simulink model "Charge_1_V1_experiment"  (R2018b)
settings: Solver=FixedStepDiscrete  StartTime=0.0  StopTime=1  FixedStep=0.001  RelTol=1e-3
PreLoadFcn:
  | librarySetup
  | eval([bdroot,'_startup']) %Calling [modelName]_startup.m
undefined symbols (not defined in the file or in its folder): A0, A1, Car1__Authorize, Car2_Authorize, CON2, CON3, CON4, Control_Mode_In, CurrentSP, D10, D12, D13, D2, D3, D4, D5, D6, D7, D8, Free_Charge, Frequency_High_Point, Frequency_Low_Point, Frequency_Mid_high, Frequency_Mid_low, HVol_High_Point, HVol_Low_Point, HVol_Mid_high, HVol_Mid_low, HVoltage_Factor, SeconCar_ThreePhase, V_Current_five, V_Current_four, V_Current_one, V_Current_six, V_Current_three, V_Current_two, V_Frequency, V_MaxPliot, V_MinPliot, Vol_High_Point, Vol_Low_Point, Vol_Mid_high, Vol_Mid_low, Voltage_Factor, Voltage_Mode_Test
libraries: simulink x324, HANcoder_STM32_Target x30, powerlib_meascontrol x8, simulink_extras x2
(part 8 of 13)

== system Charge_1_V1_experiment/HANcoder STM32 Target - E407-STM32 algorithm/Energy Meter/Energymeter_Request/RequestMessages_Enable /Subsystem ==
  In1 : Inport
  Compare To Constant11 : simulink/Logic and Bit Operations/Compare To Constant  relop=<=  const=15  OutDataTypeStr=boolean
  Compare To Constant9 : simulink/Logic and Bit Operations/Compare To Constant  relop=>=  const=0  OutDataTypeStr=boolean
  Logical Operator : Logic  AllPortsSameDT=off  OutDataTypeStr=boolean
  Out1 : Outport
  wires:
  Logical Operator/1 -> Out1/1
  Compare To Constant9/1 -> Logical Operator/1
  Compare To Constant11/1 -> Logical Operator/2
  In1/1 -> Compare To Constant11/1, Compare To Constant9/1

== system Charge_1_V1_experiment/HANcoder STM32 Target - E407-STM32 algorithm/Energy Meter/Energymeter_Request/RequestMessages_Enable /Subsystem1 ==
  In1 : Inport
  Compare To Constant19 : simulink/Logic and Bit Operations/Compare To Constant  relop=>=  const=200  OutDataTypeStr=boolean
  Compare To Constant20 : simulink/Logic and Bit Operations/Compare To Constant  relop=<=  const=215  OutDataTypeStr=boolean
  Logical Operator2 : Logic  AllPortsSameDT=off  OutDataTypeStr=boolean
  Out1 : Outport
  wires:
  In1/1 -> Compare To Constant20/1, Compare To Constant19/1
  Compare To Constant19/1 -> Logical Operator2/1
  Compare To Constant20/1 -> Logical Operator2/2
  Logical Operator2/1 -> Out1/1

== system Charge_1_V1_experiment/HANcoder STM32 Target - E407-STM32 algorithm/Energy Meter/Energymeter_Request/RequestMessages_Enable /Subsystem2 ==
  In1 : Inport
  Compare To Constant19 : simulink/Logic and Bit Operations/Compare To Constant  relop=>=  const=400  OutDataTypeStr=boolean
  Compare To Constant20 : simulink/Logic and Bit Operations/Compare To Constant  relop=<=  const=415  OutDataTypeStr=boolean
  Logical Operator2 : Logic  AllPortsSameDT=off  OutDataTypeStr=boolean
  Out1 : Outport
  wires:
  Logical Operator2/1 -> Out1/1
  Compare To Constant20/1 -> Logical Operator2/2
  Compare To Constant19/1 -> Logical Operator2/1
  In1/1 -> Compare To Constant19/1, Compare To Constant20/1

== system Charge_1_V1_experiment/HANcoder STM32 Target - E407-STM32 algorithm/Energy Meter/Energymeter_Request/RequestMessages_Enable /Subsystem3 ==
  In1 : Inport
  Compare To Constant19 : simulink/Logic and Bit Operations/Compare To Constant  relop=>=  const=600  OutDataTypeStr=boolean
  Compare To Constant20 : simulink/Logic and Bit Operations/Compare To Constant  relop=<=  const=615  OutDataTypeStr=boolean
  Logical Operator2 : Logic  AllPortsSameDT=off  OutDataTypeStr=boolean
  Out1 : Outport
  wires:
  In1/1 -> Compare To Constant20/1, Compare To Constant19/1
  Compare To Constant19/1 -> Logical Operator2/1
  Compare To Constant20/1 -> Logical Operator2/2
  Logical Operator2/1 -> Out1/1

== system Charge_1_V1_experiment/HANcoder STM32 Target - E407-STM32 algorithm/Energy Meter/Energymeter_Request/RequestMessages_Enable /Subsystem4 ==
  In1 : Inport
  Compare To Constant19 : simulink/Logic and Bit Operations/Compare To Constant  relop=>=  const=800  OutDataTypeStr=boolean
  Compare To Constant20 : simulink/Logic and Bit Operations/Compare To Constant  relop=<=  const=815  OutDataTypeStr=boolean
  Logical Operator2 : Logic  AllPortsSameDT=off  OutDataTypeStr=boolean
  Out1 : Outport
  wires:
  Logical Operator2/1 -> Out1/1
  Compare To Constant20/1 -> Logical Operator2/2
  Compare To Constant19/1 -> Logical Operator2/1
  In1/1 -> Compare To Constant19/1, Compare To Constant20/1

== system Charge_1_V1_experiment/HANcoder STM32 Target - E407-STM32 algorithm/Energy Meter/Energymeter_Request/Voltage_meter_1/Read_Gyro1 ==
  note: 01040000000271CB
  Trigger : TriggerPort  VariantControl=Variant
  Constant : Constant  Value=hex2dec('01')  OutDataTypeStr=uint8  SampleTime=-1
  UART send : Subsystem  Tag=HANcoder_TARGET_STM32_E407  AncestorBlock=HANcoder_STM32_Target/STM32-E407/UART/UART send  mask(UART send){channel=UART2: CON PD - 8 & 9, useStatusOut=off, tsamp=-1}
      mask prompts: useStatusOut "Use status outport"; tsamp "Sample time"
      mask help:
      | Function
      | ==========
      | Transmits a byte on the UART communication interface.
      |
      | Parameters per channel
      | ======================
      | - Select channel (TX & RX)
      | - Select if the status output should be enabled.
      |
      | Inputs
      | ======
      | - The byte to send
      |
      | Outputs
      | =======
      | - When the status output is 0, the byte could not be transmitted. Probably
      |   because the transmit buffer was configured too small.
      mask init:
      | uartChannelInfoStr = sfcn_uart_send_mcb(2, channel, useStatusOut);
      settings: MoveFcn=drawLogos
      mask Help: web('sfcn_uart_send.html')
      mask TypeOptions channel: UART1: CON3 - D1 & D0 | UART2: CON PD - 8 & 9 | UART3: CON PD - 11 & 12 | UART6: UEXT - 3 & 4
      mask Display: fprintf('UART send\n%s', uartChannelInfoStr);patch([245 251 251],[8 14 2],[1 0 0]);patch([253 253 259],[14 2 8],[0 0 0.35]);
  wires:
  Constant/1 -> UART send/1(In1)

== system Charge_1_V1_experiment/HANcoder STM32 Target - E407-STM32 algorithm/Energy Meter/Energymeter_Request/Voltage_meter_1/Read_Gyro2 ==
  note: 01040000000271CB
  Trigger : TriggerPort  VariantControl=Variant
  Constant1 : Constant  Value=hex2dec('04')  OutDataTypeStr=uint8  SampleTime=-1
  UART send : Subsystem  Tag=HANcoder_TARGET_STM32_E407  AncestorBlock=HANcoder_STM32_Target/STM32-E407/UART/UART send  mask(UART send){channel=UART2: CON PD - 8 & 9, useStatusOut=off, tsamp=-1}
      mask prompts: useStatusOut "Use status outport"; tsamp "Sample time"
      mask help:
      | Function
      | ==========
      | Transmits a byte on the UART communication interface.
      |
      | Parameters per channel
      | ======================
      | - Select channel (TX & RX)
      | - Select if the status output should be enabled.
      |
      | Inputs
      | ======
      | - The byte to send
      |
      | Outputs
      | =======
      | - When the status output is 0, the byte could not be transmitted. Probably
      |   because the transmit buffer was configured too small.
      mask init:
      | uartChannelInfoStr = sfcn_uart_send_mcb(2, channel, useStatusOut);
      settings: MoveFcn=drawLogos
      mask Help: web('sfcn_uart_send.html')
      mask TypeOptions channel: UART1: CON3 - D1 & D0 | UART2: CON PD - 8 & 9 | UART3: CON PD - 11 & 12 | UART6: UEXT - 3 & 4
      mask Display: fprintf('UART send\n%s', uartChannelInfoStr);patch([245 251 251],[8 14 2],[1 0 0]);patch([253 253 259],[14 2 8],[0 0 0.35]);
  wires:
  Constant1/1 -> UART send/1(In1)

== system Charge_1_V1_experiment/HANcoder STM32 Target - E407-STM32 algorithm/Energy Meter/Energymeter_Request/Voltage_meter_1/Read_Gyro3 ==
  note: 01040000000271CB
  Trigger : TriggerPort  VariantControl=Variant
  Constant2 : Constant  Value=hex2dec('00')  OutDataTypeStr=uint8  SampleTime=-1
  UART send : Subsystem  Tag=HANcoder_TARGET_STM32_E407  AncestorBlock=HANcoder_STM32_Target/STM32-E407/UART/UART send  mask(UART send){channel=UART2: CON PD - 8 & 9, useStatusOut=off, tsamp=-1}
      mask prompts: useStatusOut "Use status outport"; tsamp "Sample time"
      mask help:
      | Function
      | ==========
      | Transmits a byte on the UART communication interface.
      |
      | Parameters per channel
      | ======================
      | - Select channel (TX & RX)
      | - Select if the status output should be enabled.
      |
      | Inputs
      | ======
      | - The byte to send
      |
      | Outputs
      | =======
      | - When the status output is 0, the byte could not be transmitted. Probably
      |   because the transmit buffer was configured too small.
      mask init:
      | uartChannelInfoStr = sfcn_uart_send_mcb(2, channel, useStatusOut);
      settings: MoveFcn=drawLogos
      mask Help: web('sfcn_uart_send.html')
      mask TypeOptions channel: UART1: CON3 - D1 & D0 | UART2: CON PD - 8 & 9 | UART3: CON PD - 11 & 12 | UART6: UEXT - 3 & 4
      mask Display: fprintf('UART send\n%s', uartChannelInfoStr);patch([245 251 251],[8 14 2],[1 0 0]);patch([253 253 259],[14 2 8],[0 0 0.35]);
  wires:
  Constant2/1 -> UART send/1(In1)

== system Charge_1_V1_experiment/HANcoder STM32 Target - E407-STM32 algorithm/Energy Meter/Energymeter_Request/Voltage_meter_1/Read_Gyro4 ==
  note: 01040000000271CB
  Trigger : TriggerPort  VariantControl=Variant
  Constant4 : Constant  Value=hex2dec('00')  OutDataTypeStr=uint8  SampleTime=-1
  UART send : Subsystem  Tag=HANcoder_TARGET_STM32_E407  AncestorBlock=HANcoder_STM32_Target/STM32-E407/UART/UART send  mask(UART send){channel=UART2: CON PD - 8 & 9, useStatusOut=off, tsamp=-1}
      mask prompts: useStatusOut "Use status outport"; tsamp "Sample time"
      mask help:
      | Function
      | ==========
      | Transmits a byte on the UART communication interface.
      |
      | Parameters per channel
      | ======================
      | - Select channel (TX & RX)
      | - Select if the status output should be enabled.
      |
      | Inputs
      | ======
      | - The byte to send
      |
      | Outputs
      | =======
      | - When the status output is 0, the byte could not be transmitted. Probably
      |   because the transmit buffer was configured too small.
      mask init:
      | uartChannelInfoStr = sfcn_uart_send_mcb(2, channel, useStatusOut);
      settings: MoveFcn=drawLogos
      mask Help: web('sfcn_uart_send.html')
      mask TypeOptions channel: UART1: CON3 - D1 & D0 | UART2: CON PD - 8 & 9 | UART3: CON PD - 11 & 12 | UART6: UEXT - 3 & 4
      mask Display: fprintf('UART send\n%s', uartChannelInfoStr);patch([245 251 251],[8 14 2],[1 0 0]);patch([253 253 259],[14 2 8],[0 0 0.35]);
  wires:
  Constant4/1 -> UART send/1(In1)

== system Charge_1_V1_experiment/HANcoder STM32 Target - E407-STM32 algorithm/Energy Meter/Energymeter_Request/Voltage_meter_1/Read_Gyro5 ==
  note: 01040000000271CB
  Trigger : TriggerPort  VariantControl=Variant
  Constant5 : Constant  Value=hex2dec('00')  OutDataTypeStr=uint8  SampleTime=-1
  UART send : Subsystem  Tag=HANcoder_TARGET_STM32_E407  AncestorBlock=HANcoder_STM32_Target/STM32-E407/UART/UART send  mask(UART send){channel=UART2: CON PD - 8 & 9, useStatusOut=off, tsamp=-1}
      mask prompts: useStatusOut "Use status outport"; tsamp "Sample time"
      mask help:
      | Function
      | ==========
      | Transmits a byte on the UART communication interface.
      |
      | Parameters per channel
      | ======================
      | - Select channel (TX & RX)
      | - Select if the status output should be enabled.
      |
      | Inputs
      | ======
      | - The byte to send
      |
      | Outputs
      | =======
      | - When the status output is 0, the byte could not be transmitted. Probably
      |   because the transmit buffer was configured too small.
      mask init:
      | uartChannelInfoStr = sfcn_uart_send_mcb(2, channel, useStatusOut);
      settings: MoveFcn=drawLogos
      mask Help: web('sfcn_uart_send.html')
      mask TypeOptions channel: UART1: CON3 - D1 & D0 | UART2: CON PD - 8 & 9 | UART3: CON PD - 11 & 12 | UART6: UEXT - 3 & 4
      mask Display: fprintf('UART send\n%s', uartChannelInfoStr);patch([245 251 251],[8 14 2],[1 0 0]);patch([253 253 259],[14 2 8],[0 0 0.35]);
  wires:
  Constant5/1 -> UART send/1(In1)

== system Charge_1_V1_experiment/HANcoder STM32 Target - E407-STM32 algorithm/Energy Meter/Energymeter_Request/Voltage_meter_1/Read_Gyro6 ==
  note: 01040000000271CB
  Trigger : TriggerPort  VariantControl=Variant
  Constant6 : Constant  Value=hex2dec('06')  OutDataTypeStr=uint8  SampleTime=-1
  Terminator2 : Terminator
  UART send : Subsystem  Tag=HANcoder_TARGET_STM32_E407  AncestorBlock=HANcoder_STM32_Target/STM32-E407/UART/UART send  mask(UART send){channel=UART2: CON PD - 8 & 9, useStatusOut=off, tsamp=-1}
      mask prompts: useStatusOut "Use status outport"; tsamp "Sample time"
      mask help:
      | Function
      | ==========
      | Transmits a byte on the UART communication interface.
      |
      | Parameters per channel
      | ======================
      | - Select channel (TX & RX)
      | - Select if the status output should be enabled.
      |
      | Inputs
      | ======
      | - The byte to send
      |
      | Outputs
      | =======
      | - When the status output is 0, the byte could not be transmitted. Probably
      |   because the transmit buffer was configured too small.
      mask init:
      | uartChannelInfoStr = sfcn_uart_send_mcb(2, channel, useStatusOut);
      settings: MoveFcn=drawLogos
      mask Help: web('sfcn_uart_send.html')
      mask TypeOptions channel: UART1: CON3 - D1 & D0 | UART2: CON PD - 8 & 9 | UART3: CON PD - 11 & 12 | UART6: UEXT - 3 & 4
      mask Display: fprintf('UART send\n%s', uartChannelInfoStr);patch([245 251 251],[8 14 2],[1 0 0]);patch([253 253 259],[14 2 8],[0 0 0.35]);
  wires:
  Constant6/1 -> UART send/1(In1)

== system Charge_1_V1_experiment/HANcoder STM32 Target - E407-STM32 algorithm/Energy Meter/Energymeter_Request/Voltage_meter_1/Read_Gyro7 ==
  note: 01040000000271CB
  Trigger : TriggerPort  VariantControl=Variant
  Constant1 : Constant  Value=hex2dec('71')  OutDataTypeStr=uint8  SampleTime=-1
  Constant3 : Constant  Value=hex2dec('70')  OutDataTypeStr=uint8  SampleTime=-1
  UART send : Subsystem  Tag=HANcoder_TARGET_STM32_E407  AncestorBlock=HANcoder_STM32_Target/STM32-E407/UART/UART send  mask(UART send){channel=UART2: CON PD - 8 & 9, useStatusOut=off, tsamp=-1}
      mask prompts: useStatusOut "Use status outport"; tsamp "Sample time"
      mask help:
      | Function
      | ==========
      | Transmits a byte on the UART communication interface.
      |
      | Parameters per channel
      | ======================
      | - Select channel (TX & RX)
      | - Select if the status output should be enabled.
      |
      | Inputs
      | ======
      | - The byte to send
      |
      | Outputs
      | =======
      | - When the status output is 0, the byte could not be transmitted. Probably
      |   because the transmit buffer was configured too small.
      mask init:
      | uartChannelInfoStr = sfcn_uart_send_mcb(2, channel, useStatusOut);
      settings: MoveFcn=drawLogos
      mask Help: web('sfcn_uart_send.html')
      mask TypeOptions channel: UART1: CON3 - D1 & D0 | UART2: CON PD - 8 & 9 | UART3: CON PD - 11 & 12 | UART6: UEXT - 3 & 4
      mask Display: fprintf('UART send\n%s', uartChannelInfoStr);patch([245 251 251],[8 14 2],[1 0 0]);patch([253 253 259],[14 2 8],[0 0 0.35]);
  wires:
  Constant3/1 -> UART send/1(In1)

== system Charge_1_V1_experiment/HANcoder STM32 Target - E407-STM32 algorithm/Energy Meter/Energymeter_Request/Voltage_meter_1/Read_Gyro8 ==
  note: 01040000000271CB
  Trigger : TriggerPort  VariantControl=Variant
  Constant1 : Constant  Value=hex2dec('CB')  OutDataTypeStr=uint8  SampleTime=-1
  Constant7 : Constant  Value=hex2dec('08')  OutDataTypeStr=uint8  SampleTime=-1
  UART send : Subsystem  Tag=HANcoder_TARGET_STM32_E407  AncestorBlock=HANcoder_STM32_Target/STM32-E407/UART/UART send  mask(UART send){channel=UART2: CON PD - 8 & 9, useStatusOut=off, tsamp=-1}
      mask prompts: useStatusOut "Use status outport"; tsamp "Sample time"
      mask help:
      | Function
      | ==========
      | Transmits a byte on the UART communication interface.
      |
      | Parameters per channel
      | ======================
      | - Select channel (TX & RX)
      | - Select if the status output should be enabled.
      |
      | Inputs
      | ======
      | - The byte to send
      |
      | Outputs
      | =======
      | - When the status output is 0, the byte could not be transmitted. Probably
      |   because the transmit buffer was configured too small.
      mask init:
      | uartChannelInfoStr = sfcn_uart_send_mcb(2, channel, useStatusOut);
      settings: MoveFcn=drawLogos
      mask Help: web('sfcn_uart_send.html')
      mask TypeOptions channel: UART1: CON3 - D1 & D0 | UART2: CON PD - 8 & 9 | UART3: CON PD - 11 & 12 | UART6: UEXT - 3 & 4
      mask Display: fprintf('UART send\n%s', uartChannelInfoStr);patch([245 251 251],[8 14 2],[1 0 0]);patch([253 253 259],[14 2 8],[0 0 0.35]);
  wires:
  Constant7/1 -> UART send/1(In1)

== system Charge_1_V1_experiment/HANcoder STM32 Target - E407-STM32 algorithm/Energy Meter/Energymeter_Request/Voltage_meter_2/Read_Gyro1 ==
  note: 01040000000271CB
  Trigger : TriggerPort  VariantControl=Variant
  Constant : Constant  Value=hex2dec('02')  OutDataTypeStr=uint8  SampleTime=-1
  UART send : Subsystem  Tag=HANcoder_TARGET_STM32_E407  AncestorBlock=HANcoder_STM32_Target/STM32-E407/UART/UART send  mask(UART send){channel=UART2: CON PD - 8 & 9, useStatusOut=off, tsamp=-1}
      mask prompts: useStatusOut "Use status outport"; tsamp "Sample time"
      mask help:
      | Function
      | ==========
      | Transmits a byte on the UART communication interface.
      |
      | Parameters per channel
      | ======================
      | - Select channel (TX & RX)
      | - Select if the status output should be enabled.
      |
      | Inputs
      | ======
      | - The byte to send
      |
      | Outputs
      | =======
      | - When the status output is 0, the byte could not be transmitted. Probably
      |   because the transmit buffer was configured too small.
      mask init:
      | uartChannelInfoStr = sfcn_uart_send_mcb(2, channel, useStatusOut);
      settings: MoveFcn=drawLogos
      mask Help: web('sfcn_uart_send.html')
      mask TypeOptions channel: UART1: CON3 - D1 & D0 | UART2: CON PD - 8 & 9 | UART3: CON PD - 11 & 12 | UART6: UEXT - 3 & 4
      mask Display: fprintf('UART send\n%s', uartChannelInfoStr);patch([245 251 251],[8 14 2],[1 0 0]);patch([253 253 259],[14 2 8],[0 0 0.35]);
  wires:
  Constant/1 -> UART send/1(In1)

== system Charge_1_V1_experiment/HANcoder STM32 Target - E407-STM32 algorithm/Energy Meter/Energymeter_Request/Voltage_meter_2/Read_Gyro2 ==
  note: 01040000000271CB
  Trigger : TriggerPort  VariantControl=Variant
  Constant1 : Constant  Value=hex2dec('04')  OutDataTypeStr=uint8  SampleTime=-1
  UART send : Subsystem  Tag=HANcoder_TARGET_STM32_E407  AncestorBlock=HANcoder_STM32_Target/STM32-E407/UART/UART send  mask(UART send){channel=UART2: CON PD - 8 & 9, useStatusOut=off, tsamp=-1}
      mask prompts: useStatusOut "Use status outport"; tsamp "Sample time"
      mask help:
      | Function
      | ==========
      | Transmits a byte on the UART communication interface.
      |
      | Parameters per channel
      | ======================
      | - Select channel (TX & RX)
      | - Select if the status output should be enabled.
      |
      | Inputs
      | ======
      | - The byte to send
      |
      | Outputs
      | =======
      | - When the status output is 0, the byte could not be transmitted. Probably
      |   because the transmit buffer was configured too small.
      mask init:
      | uartChannelInfoStr = sfcn_uart_send_mcb(2, channel, useStatusOut);
      settings: MoveFcn=drawLogos
      mask Help: web('sfcn_uart_send.html')
      mask TypeOptions channel: UART1: CON3 - D1 & D0 | UART2: CON PD - 8 & 9 | UART3: CON PD - 11 & 12 | UART6: UEXT - 3 & 4
      mask Display: fprintf('UART send\n%s', uartChannelInfoStr);patch([245 251 251],[8 14 2],[1 0 0]);patch([253 253 259],[14 2 8],[0 0 0.35]);
  wires:
  Constant1/1 -> UART send/1(In1)

== system Charge_1_V1_experiment/HANcoder STM32 Target - E407-STM32 algorithm/Energy Meter/Energymeter_Request/Voltage_meter_2/Read_Gyro3 ==
  note: 01040000000271CB
  Trigger : TriggerPort  VariantControl=Variant
  Constant2 : Constant  Value=hex2dec('00')  OutDataTypeStr=uint8  SampleTime=-1
  UART send : Subsystem  Tag=HANcoder_TARGET_STM32_E407  AncestorBlock=HANcoder_STM32_Target/STM32-E407/UART/UART send  mask(UART send){channel=UART2: CON PD - 8 & 9, useStatusOut=off, tsamp=-1}
      mask prompts: useStatusOut "Use status outport"; tsamp "Sample time"
      mask help:
      | Function
      | ==========
      | Transmits a byte on the UART communication interface.
      |
      | Parameters per channel
      | ======================
      | - Select channel (TX & RX)
      | - Select if the status output should be enabled.
      |
      | Inputs
      | ======
      | - The byte to send
      |
      | Outputs
      | =======
      | - When the status output is 0, the byte could not be transmitted. Probably
      |   because the transmit buffer was configured too small.
      mask init:
      | uartChannelInfoStr = sfcn_uart_send_mcb(2, channel, useStatusOut);
      settings: MoveFcn=drawLogos
      mask Help: web('sfcn_uart_send.html')
      mask TypeOptions channel: UART1: CON3 - D1 & D0 | UART2: CON PD - 8 & 9 | UART3: CON PD - 11 & 12 | UART6: UEXT - 3 & 4
      mask Display: fprintf('UART send\n%s', uartChannelInfoStr);patch([245 251 251],[8 14 2],[1 0 0]);patch([253 253 259],[14 2 8],[0 0 0.35]);
  wires:
  Constant2/1 -> UART send/1(In1)

== system Charge_1_V1_experiment/HANcoder STM32 Target - E407-STM32 algorithm/Energy Meter/Energymeter_Request/Voltage_meter_2/Read_Gyro4 ==
  note: 01040000000271CB
  Trigger : TriggerPort  VariantControl=Variant
  Constant4 : Constant  Value=hex2dec('00')  OutDataTypeStr=uint8  SampleTime=-1
  UART send : Subsystem  Tag=HANcoder_TARGET_STM32_E407  AncestorBlock=HANcoder_STM32_Target/STM32-E407/UART/UART send  mask(UART send){channel=UART2: CON PD - 8 & 9, useStatusOut=off, tsamp=-1}
      mask prompts: useStatusOut "Use status outport"; tsamp "Sample time"
      mask help:
      | Function
      | ==========
      | Transmits a byte on the UART communication interface.
      |
      | Parameters per channel
      | ======================
      | - Select channel (TX & RX)
      | - Select if the status output should be enabled.
      |
      | Inputs
      | ======
      | - The byte to send
      |
      | Outputs
      | =======
      | - When the status output is 0, the byte could not be transmitted. Probably
      |   because the transmit buffer was configured too small.
      mask init:
      | uartChannelInfoStr = sfcn_uart_send_mcb(2, channel, useStatusOut);
      settings: MoveFcn=drawLogos
      mask Help: web('sfcn_uart_send.html')
      mask TypeOptions channel: UART1: CON3 - D1 & D0 | UART2: CON PD - 8 & 9 | UART3: CON PD - 11 & 12 | UART6: UEXT - 3 & 4
      mask Display: fprintf('UART send\n%s', uartChannelInfoStr);patch([245 251 251],[8 14 2],[1 0 0]);patch([253 253 259],[14 2 8],[0 0 0.35]);
  wires:
  Constant4/1 -> UART send/1(In1)

== system Charge_1_V1_experiment/HANcoder STM32 Target - E407-STM32 algorithm/Energy Meter/Energymeter_Request/Voltage_meter_2/Read_Gyro5 ==
  note: 01040000000271CB
  Trigger : TriggerPort  VariantControl=Variant
  Constant5 : Constant  Value=hex2dec('00')  OutDataTypeStr=uint8  SampleTime=-1
  UART send : Subsystem  Tag=HANcoder_TARGET_STM32_E407  AncestorBlock=HANcoder_STM32_Target/STM32-E407/UART/UART send  mask(UART send){channel=UART2: CON PD - 8 & 9, useStatusOut=off, tsamp=-1}
      mask prompts: useStatusOut "Use status outport"; tsamp "Sample time"
      mask help:
      | Function
      | ==========
      | Transmits a byte on the UART communication interface.
      |
      | Parameters per channel
      | ======================
      | - Select channel (TX & RX)
      | - Select if the status output should be enabled.
      |
      | Inputs
      | ======
      | - The byte to send
      |
      | Outputs
      | =======
      | - When the status output is 0, the byte could not be transmitted. Probably
      |   because the transmit buffer was configured too small.
      mask init:
      | uartChannelInfoStr = sfcn_uart_send_mcb(2, channel, useStatusOut);
      settings: MoveFcn=drawLogos
      mask Help: web('sfcn_uart_send.html')
      mask TypeOptions channel: UART1: CON3 - D1 & D0 | UART2: CON PD - 8 & 9 | UART3: CON PD - 11 & 12 | UART6: UEXT - 3 & 4
      mask Display: fprintf('UART send\n%s', uartChannelInfoStr);patch([245 251 251],[8 14 2],[1 0 0]);patch([253 253 259],[14 2 8],[0 0 0.35]);
  wires:
  Constant5/1 -> UART send/1(In1)

== system Charge_1_V1_experiment/HANcoder STM32 Target - E407-STM32 algorithm/Energy Meter/Energymeter_Request/Voltage_meter_2/Read_Gyro6 ==
  note: 01040000000271CB
  Trigger : TriggerPort  VariantControl=Variant
  Constant6 : Constant  Value=hex2dec('06')  OutDataTypeStr=uint8  SampleTime=-1
  Terminator2 : Terminator
  UART send : Subsystem  Tag=HANcoder_TARGET_STM32_E407  AncestorBlock=HANcoder_STM32_Target/STM32-E407/UART/UART send  mask(UART send){channel=UART2: CON PD - 8 & 9, useStatusOut=off, tsamp=-1}
      mask prompts: useStatusOut "Use status outport"; tsamp "Sample time"
      mask help:
      | Function
      | ==========
      | Transmits a byte on the UART communication interface.
      |
      | Parameters per channel
      | ======================
      | - Select channel (TX & RX)
      | - Select if the status output should be enabled.
      |
      | Inputs
      | ======
      | - The byte to send
      |
      | Outputs
      | =======
      | - When the status output is 0, the byte could not be transmitted. Probably
      |   because the transmit buffer was configured too small.
      mask init:
      | uartChannelInfoStr = sfcn_uart_send_mcb(2, channel, useStatusOut);
      settings: MoveFcn=drawLogos
      mask Help: web('sfcn_uart_send.html')
      mask TypeOptions channel: UART1: CON3 - D1 & D0 | UART2: CON PD - 8 & 9 | UART3: CON PD - 11 & 12 | UART6: UEXT - 3 & 4
      mask Display: fprintf('UART send\n%s', uartChannelInfoStr);patch([245 251 251],[8 14 2],[1 0 0]);patch([253 253 259],[14 2 8],[0 0 0.35]);
  wires:
  Constant6/1 -> UART send/1(In1)

== system Charge_1_V1_experiment/HANcoder STM32 Target - E407-STM32 algorithm/Energy Meter/Energymeter_Request/Voltage_meter_2/Read_Gyro7 ==
  note: 01040000000271CB
  Trigger : TriggerPort  VariantControl=Variant
  Constant1 : Constant  Value=hex2dec('71')  OutDataTypeStr=uint8  SampleTime=-1
  Constant3 : Constant  Value=hex2dec('70')  OutDataTypeStr=uint8  SampleTime=-1
  UART send : Subsystem  Tag=HANcoder_TARGET_STM32_E407  AncestorBlock=HANcoder_STM32_Target/STM32-E407/UART/UART send  mask(UART send){channel=UART2: CON PD - 8 & 9, useStatusOut=off, tsamp=-1}
      mask prompts: useStatusOut "Use status outport"; tsamp "Sample time"
      mask help:
      | Function
      | ==========
      | Transmits a byte on the UART communication interface.
      |
      | Parameters per channel
      | ======================
      | - Select channel (TX & RX)
      | - Select if the status output should be enabled.
      |
      | Inputs
      | ======
      | - The byte to send
      |
      | Outputs
      | =======
      | - When the status output is 0, the byte could not be transmitted. Probably
      |   because the transmit buffer was configured too small.
      mask init:
      | uartChannelInfoStr = sfcn_uart_send_mcb(2, channel, useStatusOut);
      settings: MoveFcn=drawLogos
      mask Help: web('sfcn_uart_send.html')
      mask TypeOptions channel: UART1: CON3 - D1 & D0 | UART2: CON PD - 8 & 9 | UART3: CON PD - 11 & 12 | UART6: UEXT - 3 & 4
      mask Display: fprintf('UART send\n%s', uartChannelInfoStr);patch([245 251 251],[8 14 2],[1 0 0]);patch([253 253 259],[14 2 8],[0 0 0.35]);
  wires:
  Constant3/1 -> UART send/1(In1)

== system Charge_1_V1_experiment/HANcoder STM32 Target - E407-STM32 algorithm/Energy Meter/Energymeter_Request/Voltage_meter_2/Read_Gyro8 ==
  note: 01040000000271CB
  Trigger : TriggerPort  VariantControl=Variant
  Constant1 : Constant  Value=hex2dec('CB')  OutDataTypeStr=uint8  SampleTime=-1
  Constant7 : Constant  Value=hex2dec('3B')  OutDataTypeStr=uint8  SampleTime=-1
  UART send : Subsystem  Tag=HANcoder_TARGET_STM32_E407  AncestorBlock=HANcoder_STM32_Target/STM32-E407/UART/UART send  mask(UART send){channel=UART2: CON PD - 8 & 9, useStatusOut=off, tsamp=-1}
      mask prompts: useStatusOut "Use status outport"; tsamp "Sample time"
      mask help:
      | Function
      | ==========
      | Transmits a byte on the UART communication interface.
      |
      | Parameters per channel
      | ======================
      | - Select channel (TX & RX)
      | - Select if the status output should be enabled.
      |
      | Inputs
      | ======
      | - The byte to send
      |
      | Outputs
      | =======
      | - When the status output is 0, the byte could not be transmitted. Probably
      |   because the transmit buffer was configured too small.
      mask init:
      | uartChannelInfoStr = sfcn_uart_send_mcb(2, channel, useStatusOut);
      settings: MoveFcn=drawLogos
      mask Help: web('sfcn_uart_send.html')
      mask TypeOptions channel: UART1: CON3 - D1 & D0 | UART2: CON PD - 8 & 9 | UART3: CON PD - 11 & 12 | UART6: UEXT - 3 & 4
      mask Display: fprintf('UART send\n%s', uartChannelInfoStr);patch([245 251 251],[8 14 2],[1 0 0]);patch([253 253 259],[14 2 8],[0 0 0.35]);
  wires:
  Constant7/1 -> UART send/1(In1)

== system Charge_1_V1_experiment/HANcoder STM32 Target - E407-STM32 algorithm/Partclie_SP_Receive/SP1/Read_Gyro/UART receive ==
  Level-2 M-file S-Function : M-S-Function  Tag=XECU_TARGET_STM32_E407  FunctionName=sfcn_uart_receive  Parameters=tsamp
  Term1 : Terminator
  Out1 : Outport
  wires:
  Level-2 M-file S-Function/2 -> Term1/1
  Level-2 M-file S-Function/1 -> Out1/1

== system Charge_1_V1_experiment/HANcoder STM32 Target - E407-STM32 algorithm/Partclie_SP_Receive/SP1/Read_Gyro1/UART receive ==
  Level-2 M-file S-Function : M-S-Function  Tag=XECU_TARGET_STM32_E407  FunctionName=sfcn_uart_receive  Parameters=tsamp
  Term1 : Terminator
  Out1 : Outport
  wires:
  Level-2 M-file S-Function/1 -> Out1/1
  Level-2 M-file S-Function/2 -> Term1/1

== system Charge_1_V1_experiment/HANcoder STM32 Target - E407-STM32 algorithm/Partclie_SP_Receive/SP1/Read_Gyro2/UART receive ==
  Level-2 M-file S-Function : M-S-Function  Tag=XECU_TARGET_STM32_E407  FunctionName=sfcn_uart_receive  Parameters=tsamp
  Term1 : Terminator
  Out1 : Outport
  wires:
  Level-2 M-file S-Function/2 -> Term1/1
  Level-2 M-file S-Function/1 -> Out1/1

== system Charge_1_V1_experiment/HANcoder STM32 Target - E407-STM32 algorithm/Partclie_SP_Receive/SP1/Read_Gyro3/UART receive ==
  Level-2 M-file S-Function : M-S-Function  Tag=XECU_TARGET_STM32_E407  FunctionName=sfcn_uart_receive  Parameters=tsamp
  Term1 : Terminator
  Out1 : Outport
  wires:
  Level-2 M-file S-Function/1 -> Out1/1
  Level-2 M-file S-Function/2 -> Term1/1

== system Charge_1_V1_experiment/HANcoder STM32 Target - E407-STM32 algorithm/Current_SP/Subsystem1/Fre_Control/Subsystem1/Subsystem ==
  In1 : Inport
  In2 : Inport  Port=2
  In3 : Inport  Port=3
  In4 : Inport  Port=4
  In5 : Inport  Port=5
  In6 : Inport  Port=6
  In7 : Inport  Port=7
  In8 : Inport  Port=8
  Constant10 : Constant  Value=5  OutDataTypeStr=single  SampleTime=-1
  Constant6 : Constant  OutDataTypeStr=single  SampleTime=-1
  Constant7 : Constant  Value=2  OutDataTypeStr=single  SampleTime=-1
  Constant8 : Constant  Value=3  OutDataTypeStr=single  SampleTime=-1
  Constant9 : Constant  Value=4  OutDataTypeStr=single  SampleTime=-1
  Logical Operator : Logic  AllPortsSameDT=off  OutDataTypeStr=boolean
  Logical Operator1 : Logic  AllPortsSameDT=off  OutDataTypeStr=boolean
  Logical Operator2 : Logic  AllPortsSameDT=off  OutDataTypeStr=boolean
  Switch{,1..4} (5 alike) : Switch  Criteria=u2 > Threshold
  Out1 : Outport
  wires:
  Constant6/1 -> Switch/1, Switch/3
  In7/1 -> Logical Operator2/2
  In6/1 -> Logical Operator2/1
  In3/1 -> Logical Operator/2
  In5/1 -> Logical Operator1/2
  In2/1 -> Logical Operator/1
  In4/1 -> Logical Operator1/1
  Logical Operator1/1 -> Switch2/2
  In1/1 -> Switch/2
  Switch1/1 -> Switch2/3
  Constant9/1 -> Switch3/1
  Switch4/1 -> Out1/1
  In8/1 -> Switch4/2
  Logical Operator/1 -> Switch1/2
  Switch/1 -> Switch1/3
  Constant7/1 -> Switch1/1
  Constant10/1 -> Switch4/1
  Constant8/1 -> Switch2/1
  Switch2/1 -> Switch3/3
  Switch3/1 -> Switch4/3
  Logical Operator2/1 -> Switch3/2

== system Charge_1_V1_experiment/HANcoder STM32 Target - E407-STM32 algorithm/Current_SP/Subsystem1/Voltage_Control/1phase/16A ==
  Vol : Inport
  Add : Sum
  Add{1..2,4..5} (4 alike) : Sum  Inputs=+-
  Add3 : Sum
  Constant : Constant  Value=11  OutDataTypeStr=single  SampleTime=-1
  Constant1 : Constant  Value=6  OutDataTypeStr=single  SampleTime=-1
  Constant2 : Constant  Value=6  OutDataTypeStr=single  SampleTime=-1
  Constant3 : Constant  Value=Vol_Low_Point  OutDataTypeStr=single  SampleTime=-1
  Constant4 : Constant  Value=16  OutDataTypeStr=single  SampleTime=-1
  Constant5 : Constant  Value=Vol_Mid_high  OutDataTypeStr=single  SampleTime=-1
  Gain : Gain  Gain=Voltage_Factor
  Gain1 : Gain  Gain=Voltage_Factor
  Product : Product
  Product1 : Product
  Out1 : Outport
  Out2 : Outport  Port=2
  Out3 : Outport  Port=3
  wires:
  Constant1/1 -> Add/2
  Add4/1 -> Product1/1
  Add1/1 -> Product/1
  Constant2/1 -> Add1/2
  Constant/1 -> Out2/1, Add1/1, Add4/2, Add3/2
  Product/1 -> Gain/1
  Constant5/1 -> Add5/2
  Constant3/1 -> Add2/2
  Add2/1 -> Product/2
  Product1/1 -> Gain1/1
  Add5/1 -> Product1/2
  Add/1 -> Out1/1
  Add3/1 -> Out3/1
  Constant4/1 -> Add4/1
  Vol/1 -> Add5/1, Add2/1
  Gain/1 -> Add/1
  Gain1/1 -> Add3/1

== system Charge_1_V1_experiment/HANcoder STM32 Target - E407-STM32 algorithm/Current_SP/Subsystem1/Voltage_Control/1phase/32Acar ==
  Vol_in : Inport
  Add : Sum
  Add{1..2,4..5} (4 alike) : Sum  Inputs=+-
  Add3 : Sum
  Constant : Constant  Value=19  OutDataTypeStr=single  SampleTime=-1
  Constant1 : Constant  Value=6  OutDataTypeStr=single  SampleTime=-1
  Constant2 : Constant  Value=6  OutDataTypeStr=single  SampleTime=-1
  Constant3 : Constant  Value=Vol_Low_Point  OutDataTypeStr=single  SampleTime=-1
  Constant4 : Constant  Value=32  OutDataTypeStr=single  SampleTime=-1
  Constant5 : Constant  Value=Vol_Mid_high  OutDataTypeStr=single  SampleTime=-1
  Gain : Gain  Gain=Voltage_Factor
  Gain1 : Gain  Gain=Voltage_Factor
  Product : Product
  Product1 : Product
  Out1 : Outport
  Out2 : Outport  Port=2
  Out3 : Outport  Port=3
  wires:
  Vol_in/1 -> Add5/1, Add2/1
  Constant4/1 -> Add4/1
  Add3/1 -> Out3/1
  Add/1 -> Out1/1
  Add5/1 -> Product1/2
  Product1/1 -> Gain1/1
  Add2/1 -> Product/2
  Constant3/1 -> Add2/2
  Constant5/1 -> Add5/2
  Product/1 -> Gain/1
  Constant/1 -> Out2/1, Add1/1, Add3/2, Add4/2
  Constant2/1 -> Add1/2
  Add1/1 -> Product/1
  Add4/1 -> Product1/1
  Constant1/1 -> Add/2
  Gain/1 -> Add/1
  Gain1/1 -> Add3/1

== system Charge_1_V1_experiment/HANcoder STM32 Target - E407-STM32 algorithm/Current_SP/Subsystem1/Voltage_Control/1phase/Subsystem ==
  In1 : Inport
  In2 : Inport  Port=2
  In3 : Inport  Port=3
  In4 : Inport  Port=4
  Compare To Constant : simulink/Logic and Bit Operations/Compare To Constant  relop=<  const=Vol_Low_Point  OutDataTypeStr=boolean
  Compare To Constant1 : simulink/Logic and Bit Operations/Compare To Constant  relop=>=  const=Vol_Low_Point  OutDataTypeStr=boolean
  Compare To Constant2 : simulink/Logic and Bit Operations/Compare To Constant  relop=<  const=Vol_Mid_low  OutDataTypeStr=boolean
  Compare To Constant3 : simulink/Logic and Bit Operations/Compare To Constant  relop=>=  const=Vol_Mid_low  OutDataTypeStr=boolean
  Compare To Constant4 : simulink/Logic and Bit Operations/Compare To Constant  relop=<  const=Vol_Mid_high  OutDataTypeStr=boolean
  Compare To Constant5 : simulink/Logic and Bit Operations/Compare To Constant  relop=>=  const=Vol_Mid_high  OutDataTypeStr=boolean
  Compare To Constant6 : simulink/Logic and Bit Operations/Compare To Constant  relop=<=  const=Vol_High_Point  OutDataTypeStr=boolean
  Compare To Constant7 : simulink/Logic and Bit Operations/Compare To Constant  relop=>  const=Vol_High_Point  OutDataTypeStr=boolean
  Constant : Constant  Value=0  OutDataTypeStr=single  SampleTime=-1
  Constant4 : Constant  Value=0  OutDataTypeStr=single  SampleTime=-1
  Multiport Switch : MultiPortSwitch  Inputs=5
  Subsystem : Subsystem
  Out1 : Outport
  wires:
  In1/1 -> Compare To Constant/1, Compare To Constant1/1, Compare To Constant2/1, Compare To Constant3/1, Compare To Constant4/1, Compare To Constant5/1, Compare To Constant7/1, Compare To Constant6/1
  Subsystem/1(Out1) -> Multiport Switch/1
  Constant/1 -> Multiport Switch/2
  Constant4/1 -> Multiport Switch/6
  Multiport Switch/1 -> Out1/1
  Compare To Constant/1 -> Subsystem/1(In1)
  Compare To Constant1/1 -> Subsystem/2(In2)
  Compare To Constant2/1 -> Subsystem/3(In3)
  Compare To Constant3/1 -> Subsystem/4(In4)
  Compare To Constant4/1 -> Subsystem/5(In5)
  Compare To Constant5/1 -> Subsystem/6(In6)
  Compare To Constant6/1 -> Subsystem/7(In7)
  Compare To Constant7/1 -> Subsystem/8(In8)
  In2/1 -> Multiport Switch/3
  In3/1 -> Multiport Switch/4
  In4/1 -> Multiport Switch/5

== system Charge_1_V1_experiment/HANcoder STM32 Target - E407-STM32 algorithm/Current_SP/Subsystem1/Voltage_Control/3phase/16A ==
  note: Voltage_Factor = the percent change in range of voltage
  Vol : Inport
  Add : Sum
  Add{1..2,4..5} (4 alike) : Sum  Inputs=+-
  Add3 : Sum
  Constant : Constant  Value=11  OutDataTypeStr=single  SampleTime=-1
  Constant1 : Constant  Value=6  OutDataTypeStr=single  SampleTime=-1
  Constant2 : Constant  Value=6  OutDataTypeStr=single  SampleTime=-1
  Constant3 : Constant  Value=HVol_Low_Point  OutDataTypeStr=single  SampleTime=-1
  Constant4 : Constant  Value=16  OutDataTypeStr=single  SampleTime=-1
  Constant5 : Constant  Value=HVol_Mid_high  OutDataTypeStr=single  SampleTime=-1
  Gain : Gain  Gain=HVoltage_Factor
  Gain1 : Gain  Gain=HVoltage_Factor
  Product : Product
  Product1 : Product
  Out1 : Outport
  Out2 : Outport  Port=2
  Out3 : Outport  Port=3
  wires:
  Gain1/1 -> Add3/1
  Gain/1 -> Add/1
  Vol/1 -> Add2/1, Add5/1
  Constant4/1 -> Add4/1
  Add3/1 -> Out3/1
  Add/1 -> Out1/1
  Add5/1 -> Product1/2
  Product1/1 -> Gain1/1
  Add2/1 -> Product/2
  Constant3/1 -> Add2/2
  Constant5/1 -> Add5/2
  Product/1 -> Gain/1
  Constant/1 -> Add3/2, Add4/2, Add1/1, Out2/1
  Constant2/1 -> Add1/2
  Add1/1 -> Product/1
  Add4/1 -> Product1/1
  Constant1/1 -> Add/2

== system Charge_1_V1_experiment/HANcoder STM32 Target - E407-STM32 algorithm/Current_SP/Subsystem1/Voltage_Control/3phase/32Acar ==
  Vol_in : Inport
  Add : Sum
  Add{1..2,4..5} (4 alike) : Sum  Inputs=+-
  Add3 : Sum
  Constant : Constant  Value=19  OutDataTypeStr=single  SampleTime=-1
  Constant1 : Constant  Value=6  OutDataTypeStr=single  SampleTime=-1
  Constant2 : Constant  Value=6  OutDataTypeStr=single  SampleTime=-1
  Constant3 : Constant  Value=HVol_Low_Point  OutDataTypeStr=single  SampleTime=-1
  Constant4 : Constant  Value=32  OutDataTypeStr=single  SampleTime=-1
  Constant5 : Constant  Value=HVol_Mid_high  OutDataTypeStr=single  SampleTime=-1
  Gain : Gain  Gain=HVoltage_Factor
  Gain1 : Gain  Gain=HVoltage_Factor
  Product : Product
  Product1 : Product
  Out1 : Outport
  Out2 : Outport  Port=2
  Out3 : Outport  Port=3
  wires:
  Gain1/1 -> Add3/1
  Gain/1 -> Add/1
  Constant1/1 -> Add/2
  Add4/1 -> Product1/1
  Add1/1 -> Product/1
  Constant2/1 -> Add1/2
  Constant/1 -> Add4/2, Add3/2, Add1/1, Out2/1
  Product/1 -> Gain/1
  Constant5/1 -> Add5/2
  Constant3/1 -> Add2/2
  Add2/1 -> Product/2
  Product1/1 -> Gain1/1
  Add5/1 -> Product1/2
  Add/1 -> Out1/1
  Add3/1 -> Out3/1
  Constant4/1 -> Add4/1
  Vol_in/1 -> Add2/1, Add5/1

== system Charge_1_V1_experiment/HANcoder STM32 Target - E407-STM32 algorithm/Current_SP/Subsystem1/Voltage_Control/3phase/Subsystem1 ==
  In1 : Inport
  In2 : Inport  Port=2
  In3 : Inport  Port=3
  In4 : Inport  Port=4
  Compare To Constant : simulink/Logic and Bit Operations/Compare To Constant  relop=<  const=HVol_Low_Point  OutDataTypeStr=boolean
  Compare To Constant1 : simulink/Logic and Bit Operations/Compare To Constant  relop=>=  const=HVol_Low_Point  OutDataTypeStr=boolean
  Compare To Constant2 : simulink/Logic and Bit Operations/Compare To Constant  relop=<  const=HVol_Mid_low  OutDataTypeStr=boolean
  Compare To Constant3 : simulink/Logic and Bit Operations/Compare To Constant  relop=>=  const=HVol_Mid_low  OutDataTypeStr=boolean
  Compare To Constant4 : simulink/Logic and Bit Operations/Compare To Constant  relop=<  const=HVol_Mid_high  OutDataTypeStr=boolean
  Compare To Constant5 : simulink/Logic and Bit Operations/Compare To Constant  relop=>=  const=HVol_Mid_high  OutDataTypeStr=boolean
  Compare To Constant6 : simulink/Logic and Bit Operations/Compare To Constant  relop=<=  const=HVol_High_Point  OutDataTypeStr=boolean
  Compare To Constant7 : simulink/Logic and Bit Operations/Compare To Constant  relop=>  const=HVol_High_Point  OutDataTypeStr=boolean
  Constant : Constant  Value=0  OutDataTypeStr=single  SampleTime=-1
  Constant4 : Constant  Value=0  OutDataTypeStr=single  SampleTime=-1
  Multiport Switch : MultiPortSwitch  Inputs=5
  Subsystem : Subsystem
  Out1 : Outport
  wires:
  In4/1 -> Multiport Switch/5
  In3/1 -> Multiport Switch/4
  In2/1 -> Multiport Switch/3
  Compare To Constant7/1 -> Subsystem/8(In8)
  Compare To Constant6/1 -> Subsystem/7(In7)
  Compare To Constant5/1 -> Subsystem/6(In6)
  Compare To Constant4/1 -> Subsystem/5(In5)
  Compare To Constant3/1 -> Subsystem/4(In4)
  Compare To Constant2/1 -> Subsystem/3(In3)
  Compare To Constant1/1 -> Subsystem/2(In2)
  Compare To Constant/1 -> Subsystem/1(In1)
  Multiport Switch/1 -> Out1/1
  Constant4/1 -> Multiport Switch/6
  Constant/1 -> Multiport Switch/2
  Subsystem/1(Out1) -> Multiport Switch/1
  In1/1 -> Compare To Constant6/1, Compare To Constant7/1, Compare To Constant5/1, Compare To Constant4/1, Compare To Constant3/1, Compare To Constant2/1, Compare To Constant1/1, Compare To Constant/1

== system Charge_1_V1_experiment/HANcoder STM32 Target - E407-STM32 algorithm/Current_SP/Subsystem2/Frquency_Control/Subsystem/Subsystem ==
  In1 : Inport
  In2 : Inport  Port=2
  In3 : Inport  Port=3
  In4 : Inport  Port=4
  In5 : Inport  Port=5
  In6 : Inport  Port=6
  In7 : Inport  Port=7
  In8 : Inport  Port=8
  Constant10 : Constant  Value=5  OutDataTypeStr=single  SampleTime=-1
  Constant6 : Constant  OutDataTypeStr=single  SampleTime=-1
  Constant7 : Constant  Value=2  OutDataTypeStr=single  SampleTime=-1
  Constant8 : Constant  Value=3  OutDataTypeStr=single  SampleTime=-1
  Constant9 : Constant  Value=4  OutDataTypeStr=single  SampleTime=-1
  Logical Operator : Logic  AllPortsSameDT=off  OutDataTypeStr=boolean
  Logical Operator1 : Logic  AllPortsSameDT=off  OutDataTypeStr=boolean
  Logical Operator2 : Logic  AllPortsSameDT=off  OutDataTypeStr=boolean
  Switch{,1..4} (5 alike) : Switch  Criteria=u2 > Threshold
  Out1 : Outport
  wires:
  Constant6/1 -> Switch/1, Switch/3
  In7/1 -> Logical Operator2/2
  In6/1 -> Logical Operator2/1
  In3/1 -> Logical Operator/2
  In5/1 -> Logical Operator1/2
  In2/1 -> Logical Operator/1
  In4/1 -> Logical Operator1/1
  Logical Operator1/1 -> Switch2/2
  In1/1 -> Switch/2
  Switch1/1 -> Switch2/3
  Constant9/1 -> Switch3/1
  Switch4/1 -> Out1/1
  In8/1 -> Switch4/2
  Logical Operator/1 -> Switch1/2
  Switch/1 -> Switch1/3
  Constant7/1 -> Switch1/1
  Constant10/1 -> Switch4/1
  Constant8/1 -> Switch2/1
  Switch2/1 -> Switch3/3
  Switch3/1 -> Switch4/3
  Logical Operator2/1 -> Switch3/2

== system Charge_1_V1_experiment/HANcoder STM32 Target - E407-STM32 algorithm/Current_SP/Subsystem2/Voltage_Control/1phase/16A ==
  Vol : Inport
  Add : Sum
  Add{1..2,4..5} (4 alike) : Sum  Inputs=+-
  Add3 : Sum
  Constant : Constant  Value=11  OutDataTypeStr=single  SampleTime=-1
  Constant1 : Constant  Value=6  OutDataTypeStr=single  SampleTime=-1
  Constant2 : Constant  Value=6  OutDataTypeStr=single  SampleTime=-1
  Constant3 : Constant  Value=Vol_Low_Point  OutDataTypeStr=single  SampleTime=-1
  Constant4 : Constant  Value=16  OutDataTypeStr=single  SampleTime=-1
  Constant5 : Constant  Value=Vol_Mid_high  OutDataTypeStr=single  SampleTime=-1
  Gain : Gain  Gain=Voltage_Factor
  Gain1 : Gain  Gain=Voltage_Factor
  Product : Product
  Product1 : Product
  Out1 : Outport
  Out2 : Outport  Port=2
  Out3 : Outport  Port=3
  wires:
  Constant1/1 -> Add/2
  Add4/1 -> Product1/1
  Add1/1 -> Product/1
  Constant2/1 -> Add1/2
  Constant/1 -> Out2/1, Add1/1, Add4/2, Add3/2
  Product/1 -> Gain/1
  Constant5/1 -> Add5/2
  Constant3/1 -> Add2/2
  Add2/1 -> Product/2
  Product1/1 -> Gain1/1
  Add5/1 -> Product1/2
  Add/1 -> Out1/1
  Add3/1 -> Out3/1
  Constant4/1 -> Add4/1
  Vol/1 -> Add5/1, Add2/1
  Gain/1 -> Add/1
  Gain1/1 -> Add3/1

== system Charge_1_V1_experiment/HANcoder STM32 Target - E407-STM32 algorithm/Current_SP/Subsystem2/Voltage_Control/1phase/32Acar ==
  note: Voltage_Factor = the percent change in range of voltage (215 245 as default for 1phase)
  Vol_in : Inport
  Add : Sum
  Add{1..2,4..5} (4 alike) : Sum  Inputs=+-
  Add3 : Sum
  Constant : Constant  Value=19  OutDataTypeStr=single  SampleTime=-1
  Constant1 : Constant  Value=6  OutDataTypeStr=single  SampleTime=-1
  Constant2 : Constant  Value=6  OutDataTypeStr=single  SampleTime=-1
  Constant3 : Constant  Value=Vol_Low_Point  OutDataTypeStr=single  SampleTime=-1
  Constant4 : Constant  Value=32  OutDataTypeStr=single  SampleTime=-1
  Constant5 : Constant  Value=Vol_Mid_high  OutDataTypeStr=single  SampleTime=-1
  Gain : Gain  Gain=Voltage_Factor
  Gain1 : Gain  Gain=Voltage_Factor
  Product : Product
  Product1 : Product
  Out1 : Outport
  Out2 : Outport  Port=2
  Out3 : Outport  Port=3
  wires:
  Vol_in/1 -> Add5/1, Add2/1
  Constant4/1 -> Add4/1
  Add3/1 -> Out3/1
  Add/1 -> Out1/1
  Add5/1 -> Product1/2
  Product1/1 -> Gain1/1
  Add2/1 -> Product/2
  Constant3/1 -> Add2/2
  Constant5/1 -> Add5/2
  Product/1 -> Gain/1
  Constant/1 -> Out2/1, Add1/1, Add3/2, Add4/2
  Constant2/1 -> Add1/2
  Add1/1 -> Product/1
  Add4/1 -> Product1/1
  Constant1/1 -> Add/2
  Gain/1 -> Add/1
  Gain1/1 -> Add3/1

== system Charge_1_V1_experiment/HANcoder STM32 Target - E407-STM32 algorithm/Current_SP/Subsystem2/Voltage_Control/1phase/Subsystem ==
  In1 : Inport
  In2 : Inport  Port=2
  In3 : Inport  Port=3
  In4 : Inport  Port=4
  Compare To Constant : simulink/Logic and Bit Operations/Compare To Constant  relop=<  const=Vol_Low_Point  OutDataTypeStr=boolean
  Compare To Constant1 : simulink/Logic and Bit Operations/Compare To Constant  relop=>=  const=Vol_Low_Point  OutDataTypeStr=boolean
  Compare To Constant2 : simulink/Logic and Bit Operations/Compare To Constant  relop=<  const=Vol_Mid_low  OutDataTypeStr=boolean
  Compare To Constant3 : simulink/Logic and Bit Operations/Compare To Constant  relop=>=  const=Vol_Mid_low  OutDataTypeStr=boolean
  Compare To Constant4 : simulink/Logic and Bit Operations/Compare To Constant  relop=<  const=Vol_Mid_high  OutDataTypeStr=boolean
  Compare To Constant5 : simulink/Logic and Bit Operations/Compare To Constant  relop=>=  const=Vol_Mid_high  OutDataTypeStr=boolean
  Compare To Constant6 : simulink/Logic and Bit Operations/Compare To Constant  relop=<=  const=Vol_High_Point  OutDataTypeStr=boolean
  Compare To Constant7 : simulink/Logic and Bit Operations/Compare To Constant  relop=>  const=Vol_High_Point  OutDataTypeStr=boolean
  Constant : Constant  Value=0  OutDataTypeStr=single  SampleTime=-1
  Constant4 : Constant  Value=0  OutDataTypeStr=single  SampleTime=-1
  Multiport Switch : MultiPortSwitch  Inputs=5
  Subsystem : Subsystem
  Out1 : Outport
  wires:
  In1/1 -> Compare To Constant/1, Compare To Constant1/1, Compare To Constant2/1, Compare To Constant3/1, Compare To Constant4/1, Compare To Constant5/1, Compare To Constant7/1, Compare To Constant6/1
  Subsystem/1(Out1) -> Multiport Switch/1
  Constant/1 -> Multiport Switch/2
  Constant4/1 -> Multiport Switch/6
  Multiport Switch/1 -> Out1/1
  Compare To Constant/1 -> Subsystem/1(In1)
  Compare To Constant1/1 -> Subsystem/2(In2)
  Compare To Constant2/1 -> Subsystem/3(In3)
  Compare To Constant3/1 -> Subsystem/4(In4)
  Compare To Constant4/1 -> Subsystem/5(In5)
  Compare To Constant5/1 -> Subsystem/6(In6)
  Compare To Constant6/1 -> Subsystem/7(In7)
  Compare To Constant7/1 -> Subsystem/8(In8)
  In2/1 -> Multiport Switch/3
  In3/1 -> Multiport Switch/4
  In4/1 -> Multiport Switch/5

== system Charge_1_V1_experiment/HANcoder STM32 Target - E407-STM32 algorithm/Current_SP/Subsystem2/Voltage_Control/3phase/16A ==
  note: Voltage_Factor = the percent change in range of voltage
  Vol : Inport
  Add : Sum
  Add{1..2,4..5} (4 alike) : Sum  Inputs=+-
  Add3 : Sum
  Constant : Constant  Value=11  OutDataTypeStr=single  SampleTime=-1
  Constant1 : Constant  Value=6  OutDataTypeStr=single  SampleTime=-1
  Constant2 : Constant  Value=6  OutDataTypeStr=single  SampleTime=-1
  Constant3 : Constant  Value=HVol_Low_Point  OutDataTypeStr=single  SampleTime=-1
  Constant4 : Constant  Value=16  OutDataTypeStr=single  SampleTime=-1
  Constant5 : Constant  Value=HVol_Mid_high  OutDataTypeStr=single  SampleTime=-1
  Gain : Gain  Gain=HVoltage_Factor
  Gain1 : Gain  Gain=HVoltage_Factor
  Product : Product
  Product1 : Product
  Out1 : Outport
  Out2 : Outport  Port=2
  Out3 : Outport  Port=3
  wires:
  Gain1/1 -> Add3/1
  Gain/1 -> Add/1
  Vol/1 -> Add2/1, Add5/1
  Constant4/1 -> Add4/1
  Add3/1 -> Out3/1
  Add/1 -> Out1/1
  Add5/1 -> Product1/2
  Product1/1 -> Gain1/1
  Add2/1 -> Product/2
  Constant3/1 -> Add2/2
  Constant5/1 -> Add5/2
  Product/1 -> Gain/1
  Constant/1 -> Add3/2, Add4/2, Add1/1, Out2/1
  Constant2/1 -> Add1/2
  Add1/1 -> Product/1
  Add4/1 -> Product1/1
  Constant1/1 -> Add/2

== system Charge_1_V1_experiment/HANcoder STM32 Target - E407-STM32 algorithm/Current_SP/Subsystem2/Voltage_Control/3phase/32Acar ==
  note: Voltage_Factor = the percent change in range of voltage
  Vol_in : Inport
  Add : Sum
  Add{1..2,4..5} (4 alike) : Sum  Inputs=+-
  Add3 : Sum
  Constant : Constant  Value=19  OutDataTypeStr=single  SampleTime=-1
  Constant1 : Constant  Value=6  OutDataTypeStr=single  SampleTime=-1
  Constant2 : Constant  Value=6  OutDataTypeStr=single  SampleTime=-1
  Constant3 : Constant  Value=HVol_Low_Point  OutDataTypeStr=single  SampleTime=-1
  Constant4 : Constant  Value=32  OutDataTypeStr=single  SampleTime=-1
  Constant5 : Constant  Value=HVol_Mid_high  OutDataTypeStr=single  SampleTime=-1
  Gain : Gain  Gain=HVoltage_Factor
  Gain1 : Gain  Gain=HVoltage_Factor
  Product : Product
  Product1 : Product
  Out1 : Outport
  Out2 : Outport  Port=2
  Out3 : Outport  Port=3
  wires:
  Gain1/1 -> Add3/1
  Gain/1 -> Add/1
  Constant1/1 -> Add/2
  Add4/1 -> Product1/1
  Add1/1 -> Product/1
  Constant2/1 -> Add1/2
  Constant/1 -> Add4/2, Add3/2, Add1/1, Out2/1
  Product/1 -> Gain/1
  Constant5/1 -> Add5/2
  Constant3/1 -> Add2/2
  Add2/1 -> Product/2
  Product1/1 -> Gain1/1
  Add5/1 -> Product1/2
  Add/1 -> Out1/1
  Add3/1 -> Out3/1
  Constant4/1 -> Add4/1
  Vol_in/1 -> Add2/1, Add5/1
